simulink library "Load_lib"  (Simulink 8.1)
settings: Solver=ode45  StartTime=0.0  StopTime=10.0  RelTol=1e-3
undefined symbols (not defined in the file): gcbh, sps_rtmsupport, Ts
libraries: powerlib x9, simulink x2, breaker_lib x1, spsPLL3phModel x1, Load_lib x1, powerlib_meascontrol x1
settings Model: Creator=re25624  LastModifiedBy=re25624

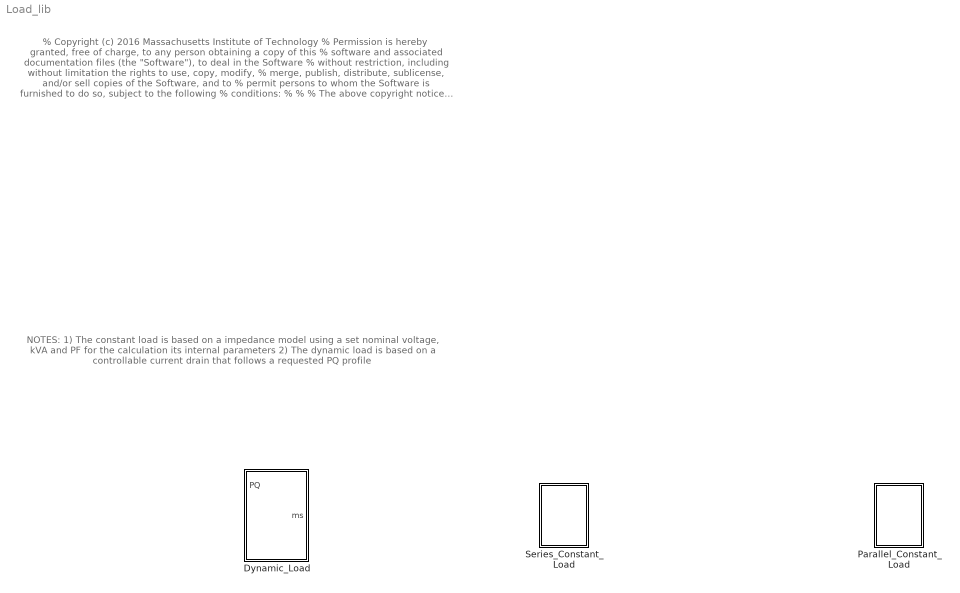
== system Load_lib ==
  note: NOTES:
      | 1) The constant load is based on a impedance model using a set nominal voltage, kVA and PF for the calculation its internal parameters
      |
      | 2) The dynamic load is based on a controllable current drain that follows a requested PQ profile
  note: % Copyright (c) 2016 Massachusetts Institute of Technology
      | % Permission is hereby granted, free of charge, to any person obtaining a copy of this
      | % software and associated documentation files (the "Software"), to deal in the Software
      | % without restriction, including without limitation the rights to use, copy, modify,
      | % merge, publish, distribute, sublicense, and/or sell copies of the Software, and to
      | % permit persons to whom the Software is furnished to do so, subject to the following
      | % conditions:
      | %
      | %
      | % The above copyright notice and this permission notice shall be included in
      | % all copies or substantial portions of the Software.
      | %
      | % THE SOFTWARE IS PROVIDED "AS IS", WITHOUT WARRANTY OF ANY KIND, EXPRESS OR IMPLIED,
      | % INCLUDING BUT NOT LIMITED TO THE WARRANTIES OF MERCHANTABILITY, FITNESS FOR A
      | % PARTICULAR PURPOSE AND NONINFRINGEMENT. IN NO EVENT SHALL THE AUTHORS OR COPYRIGHT
      | % HOLDERS BE LIABLE FOR ANY CLAIM, DAMAGES OR OTHER LIABILITY, WHETHER IN AN ACTION
      | % OF CONTRACT, TORT OR OTHERWISE, ARISING FROM, OUT OF OR IN CONNECTION WITH THE
      | % SOFTWARE OR THE USE OR OTHER DEALINGS IN THE SOFTWARE.
      | %
      | %
      | %%
  Dynamic_Load : Subsystem  mask(Dynamic load){V=460, Ts=Ts}
      mask prompts: V "VRMSLL"; Ts "Simulation Step"
      mask help:
      | The dynamic load model is based on three independent current drains (initialized using nominal voltage) following a terminal voltage and the feed-in kW and kVAr.
      |
      | The current drain of each phase is computed independently permitting unbalanced conditions in the system resulting in unbalanced consumption.
  Parallel_Constant_Load : Subsystem  mask(Static Parallel PQ Load){v=460, kVA=100, pf=0.90}
      mask prompts: v "VRMSLL"
      mask help: The static load model is based on the default Simulink parallel load model. However, a mask was created to permit parametrization using nominal voltage, apparent power, and power factor.
  Series_Constant_Load : Subsystem  mask(Static Series PQ Load){v=460, kVA=100, pf=0.90}
      mask prompts: v "VRMSLL"
      mask help: The static load model is based on the default Simulink parallel load model. However, a mask was created to permit parametrization using nominal voltage, apparent power, and power factor.

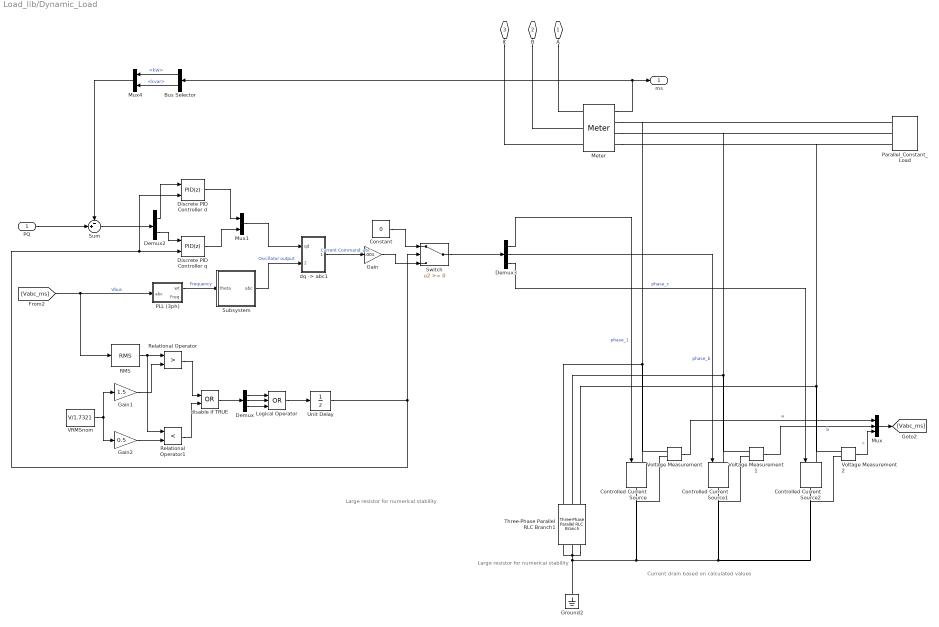
== system Load_lib/Dynamic_Load ==
  note: Large resistor for numerical stability
  note: Current drain based on calculated values
  note: Large resistor for numerical stability
  PQ : Inport
  Bus Selector : BusSelector  OutputSignals=kW,kvar
  Constant : Constant  Value=0
  Controlled Current Source : powerlib/Electrical Sources/Controlled Current Source  Initialize=on  Source_Type=AC  Amplitude=0  Phase=0  Frequency=0  Measurements=None
  Controlled Current Source1 : powerlib/Electrical Sources/Controlled Current Source  Initialize=on  Source_Type=AC  Amplitude=0  Phase=0  Frequency=0  Measurements=None
  Controlled Current Source2 : powerlib/Electrical Sources/Controlled Current Source  Initialize=on  Source_Type=AC  Amplitude=0  Phase=0  Frequency=0  Measurements=None
  Demux : Demux  Outputs=3
  Demux2 : Demux  Outputs=2
  Demux3 : Demux  Outputs=3
  Discrete PID Controller d : simulink/Continuous/PID Controller  Controller=PID  TimeDomain=Discrete-time  SampleTime=Ts  IntegratorMethod=Forward Euler  FilterMethod=Forward Euler  Form=Parallel  P=0  I=2000  D=0  N=100  InitialConditionSource=internal  InitialConditionForIntegrator=0  InitialConditionForFilter=0  ExternalReset=level  LimitOutput=off  UpperSaturationLimit=inf  LowerSaturationLimit=-inf  LinearizeAsGain=off  AntiWindupMode=none  Kb=1  TrackingMode=off  Kt=1  PParamMin=[]  PParamMax=[]  IParamMin=[]  IParamMax=[]  DParamMin=[]  DParamMax=[]  NParamMin=[]  NParamMax=[]  KbParamMin=[]  KbParamMax=[]  KtParamMin=[]  KtParamMax=[]  POutMin=[]  POutMax=[]  IOutMin=[]  IOutMax=[]  DOutMin=[]  DOutMax=[]  NOutMin=[]  NOutMax=[]  KbOutMin=[]  KbOutMax=[]  KtOutMin=[]  KtOutMax=[]  IntegratorOutMin=[]  IntegratorOutMax=[]  FilterOutMin=[]  FilterOutMax=[]  SumOutMin=[]  SumOutMax=[]  SumI1OutMin=[]  SumI1OutMax=[]  SumI2OutMin=[]  SumI2OutMax=[]  SumI3OutMin=[]  SumI3OutMax=[]  SumDOutMin=[]  SumDOutMax=[]  SaturationOutMin=[]  SaturationOutMax=[]  IntegratorContinuousStateAttributes=''  IntegratorStateMustResolveToSignalObject=off  IntegratorRTWStateStorageClass=Auto  FilterContinuousStateAttributes=''  FilterStateMustResolveToSignalObject=off  FilterRTWStateStorageClass=Auto
  Discrete PID Controller q : simulink/Continuous/PID Controller  Controller=PID  TimeDomain=Discrete-time  SampleTime=Ts  IntegratorMethod=Forward Euler  FilterMethod=Forward Euler  Form=Parallel  P=0  I=-2000  D=0  N=100  InitialConditionSource=internal  InitialConditionForIntegrator=0  InitialConditionForFilter=0  ExternalReset=level  LimitOutput=off  UpperSaturationLimit=inf  LowerSaturationLimit=-inf  LinearizeAsGain=off  AntiWindupMode=none  Kb=1  TrackingMode=off  Kt=1  PParamMin=[]  PParamMax=[]  IParamMin=[]  IParamMax=[]  DParamMin=[]  DParamMax=[]  NParamMin=[]  NParamMax=[]  KbParamMin=[]  KbParamMax=[]  KtParamMin=[]  KtParamMax=[]  POutMin=[]  POutMax=[]  IOutMin=[]  IOutMax=[]  DOutMin=[]  DOutMax=[]  NOutMin=[]  NOutMax=[]  KbOutMin=[]  KbOutMax=[]  KtOutMin=[]  KtOutMax=[]  IntegratorOutMin=[]  IntegratorOutMax=[]  FilterOutMin=[]  FilterOutMax=[]  SumOutMin=[]  SumOutMax=[]  SumI1OutMin=[]  SumI1OutMax=[]  SumI2OutMin=[]  SumI2OutMax=[]  SumI3OutMin=[]  SumI3OutMax=[]  SumDOutMin=[]  SumDOutMax=[]  SaturationOutMin=[]  SaturationOutMax=[]  IntegratorContinuousStateAttributes=''  IntegratorStateMustResolveToSignalObject=off  IntegratorRTWStateStorageClass=Auto  FilterContinuousStateAttributes=''  FilterStateMustResolveToSignalObject=off  FilterRTWStateStorageClass=Auto
  Gain : Gain  Gain=.001
  Gain1 : Gain  Gain=1.5
  Gain2 : Gain  Gain=0.5
  Ground2 : powerlib/Elements/Ground  LConnTagsString=a
  Logical Operator : Logic  Operator=OR  Inputs=3  AllPortsSameDT=off  OutDataTypeStr=boolean
  Meter : breaker_lib/Meter  Ts=Ts
  Mux : Mux  Inputs=3
  Mux1 : Mux  Inputs=2
  Mux4 : Mux  Inputs=2
  PLL (3ph) : Subsystem  DialogController=POWERSYS.PowerSysDialog  mask(PLL (3ph)){Fmin=45, Par_Init=[0, 60], ParK=[180, 5000, 1], TcD=1e-4, MaxRateChangeFreq=12, FilterCutOffFreq=25, Ts=Ts, AGC=on}
      mask prompts: Fmin "Minimum frequency (Hz):"; Par_Init "Initial inputs [ Phase (degrees), Frequency (Hz) ]:"; ParK "Regulator gains [ Kp, Ki, Kd ]:"; TcD "Time constant for derivative action (s):"; MaxRateChangeFreq "Maximum rate of change of frequency (Hz/s):"; FilterCutOffFreq "Filter cut-off frequency for frequency measurement (Hz):"; Ts "Sample time:"; AGC "Enable automatic gain control"
      mask help:
      | This Phase Locked Loop (PLL) system can be used  to synchronize on a set of variable frequency, three-phase sinusoidal signals. If the Automatic Gain Control is enabled, the input (phase error) of the PLL regulator is scaled according to the input signals magnitude.
      |
      | For optimal performance, set regulator gains [ Kp Ki  Kd ] = [ 180  3200  1 ] and check the Enable Automatic Gain Control parameter.
      |
      | Input : Vector containing the normalized three-phase signals [Va Vb Vc]
      | Output 1:  Measured frequency (Hz) = w/(2pi)
      | Output 2:  Ramp w.t varying between  0 and 2*pi, synchronized on zero crossings of the fundamental (positive-sequence) of phase A.
      mask init:
      | block=gcb;
      | [WantBlockChoice,Ts,sps] = powericon('PLL3phInit',block,Fmin,Par_Init,ParK,TcD, MaxRateChangeFreq, FilterCutOffFreq, AGC,Ts);
      | powericon('SetInternalModels','set',block,WantBlockChoice);
      settings: OpenFcn=power_openblockproxy();
      mask Help: helpview(psbhelp);
  Parallel_Constant_Load : Load_lib/Parallel_Constant_Load  v=V  kVA=5  pf=0.9
  RMS : powerlib_meascontrol/Measurements/RMS  TrueRMS=on  Freq=60  RMSInit=120  Ts=Ts
  Relational Operator : RelationalOperator  Operator=>  OutDataTypeStr=boolean
  Relational Operator1 : RelationalOperator  Operator=<  OutDataTypeStr=boolean
  Subsystem : Subsystem
  Sum : Sum  Inputs=-+|
  Switch : Switch
  Three-Phase Parallel RLC Branch1 : powerlib/Elements/Three-Phase Parallel RLC Branch  LConnTagsString=A|B|C  RConnTagsString=A|B|C  BranchType=RLC  Resistance=1e6  Inductance=inf  Capacitance=0  Measurements=None
  Unit Delay : UnitDelay  SampleTime=-1
  VRMSnom : Constant  Value=V/1.7321  SampleTime=Ts
  Voltage Measurement : powerlib/Measurements/Voltage Measurement  PhasorSimulation=off  OutputType=Complex  PSBequivalent=0
  Voltage Measurement1 : powerlib/Measurements/Voltage Measurement  PhasorSimulation=off  OutputType=Complex  PSBequivalent=0
  Voltage Measurement2 : powerlib/Measurements/Voltage Measurement  PhasorSimulation=off  OutputType=Complex  PSBequivalent=0
  disable if TRUE : Logic  Operator=OR  AllPortsSameDT=off  OutDataTypeStr=boolean
  "dq -> abc1" : Subsystem
  A : PMIOPort  Port=1  Side=Left
  B : PMIOPort  Port=2  Side=Left
  C : PMIOPort  Port=3  Side=Left
  ms : Outport
  wires:
  Voltage Measurement/1 -> Mux/1  "a"
  Voltage Measurement1/1 -> Mux/2  "b"
  Voltage Measurement2/1 -> Mux/3  "c"
  Mux/1 -> [Vabc_ms]
  Demux3/1 -> Controlled Current Source/1  "phase_1"
  Demux3/2 -> Controlled Current Source1/1  "phase_b"
  Demux3/3 -> Controlled Current Source2/1  "phase_c"
  Switch/1 -> Demux3/1
  Gain/1 -> Switch/3
  PLL (3ph)/1(wt) -> Subsystem/1(theta)  "Frequency"
  Subsystem/1(abc) -> "dq -> abc1"/2(Vabc)  "Oscillator output"
  Mux4/1 -> Sum/1
  Discrete PID Controller q/1 -> Mux1/2
  Discrete PID Controller d/1 -> Mux1/1
  Mux1/1 -> "dq -> abc1"/1(qd)
  Demux2/2 -> Discrete PID Controller q/1
  Demux2/1 -> Discrete PID Controller d/1
  Sum/1 -> Demux2/1
  "dq -> abc1"/1(abc) -> Gain/1  "Current Command_abc"
  [Vabc_ms] -> PLL (3ph)/1(abc), RMS/1  "Vbus"
  PQ/1 -> Sum/2
  RMS/1 -> Relational Operator/1, Relational Operator1/1
  VRMSnom/1 -> Gain2/1, Gain1/1
  Gain1/1 -> Relational Operator/2
  Gain2/1 -> Relational Operator1/2
  Relational Operator/1 -> disable if TRUE/1
  Relational Operator1/1 -> disable if TRUE/2
  disable if TRUE/1 -> Demux/1
  Constant/1 -> Switch/1
  Unit Delay/1 -> Discrete PID Controller q/2, Discrete PID Controller d/2, Switch/2
  Demux/1 -> Logical Operator/1
  Demux/2 -> Logical Operator/2
  Demux/3 -> Logical Operator/3
  Logical Operator/1 -> Unit Delay/1
  Bus Selector/1 -> Mux4/1  "<kW>"
  Bus Selector/2 -> Mux4/2  "<kvar>"
  Meter/1 -> ms/1, Bus Selector/1
  connections:
  Voltage Measurement/LConn1 -- Controlled Current Source/LConn1 -- Meter/RConn1 -- Parallel_Constant_Load/RConn1 -- Three-Phase Parallel RLC Branch1/RConn1
  Voltage Measurement1/LConn1 -- Controlled Current Source1/LConn1 -- Parallel_Constant_Load/RConn2 -- Meter/RConn2 -- Three-Phase Parallel RLC Branch1/RConn2
  Voltage Measurement2/LConn1 -- Controlled Current Source2/LConn1 -- Parallel_Constant_Load/RConn3 -- Meter/RConn3 -- Three-Phase Parallel RLC Branch1/RConn3
  Voltage Measurement2/LConn2 -- Controlled Current Source2/RConn1 -- Three-Phase Parallel RLC Branch1/LConn1 -- Three-Phase Parallel RLC Branch1/LConn2 -- Three-Phase Parallel RLC Branch1/LConn3 -- Ground2/LConn1 -- Voltage Measurement/LConn2 -- Controlled Current Source/RConn1 -- Voltage Measurement1/LConn2 -- Controlled Current Source1/RConn1
  A/RConn1 -- Meter/LConn1
  B/RConn1 -- Meter/LConn2
  C/RConn1 -- Meter/LConn3

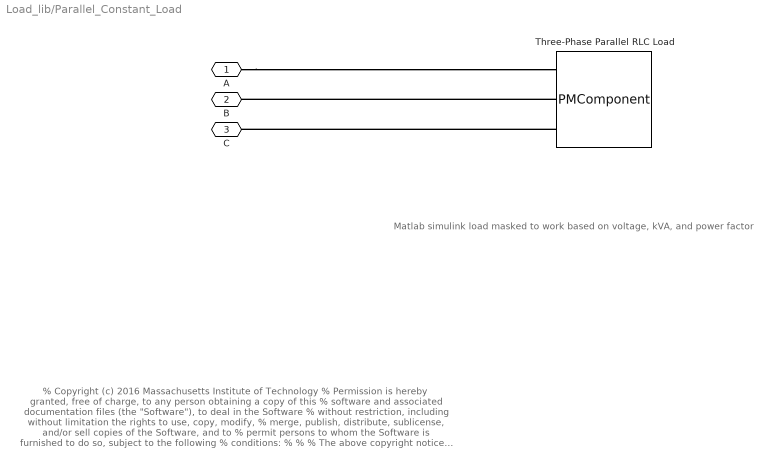
== system Load_lib/Parallel_Constant_Load ==
  note: Matlab simulink load masked to work based on voltage, kVA, and power factor
  note: % Copyright (c) 2016 Massachusetts Institute of Technology
      | % Permission is hereby granted, free of charge, to any person obtaining a copy of this
      | % software and associated documentation files (the "Software"), to deal in the Software
      | % without restriction, including without limitation the rights to use, copy, modify,
      | % merge, publish, distribute, sublicense, and/or sell copies of the Software, and to
      | % permit persons to whom the Software is furnished to do so, subject to the following
      | % conditions:
      | %
      | %
      | % The above copyright notice and this permission notice shall be included in
      | % all copies or substantial portions of the Software.
      | %
      | % THE SOFTWARE IS PROVIDED "AS IS", WITHOUT WARRANTY OF ANY KIND, EXPRESS OR IMPLIED,
      | % INCLUDING BUT NOT LIMITED TO THE WARRANTIES OF MERCHANTABILITY, FITNESS FOR A
      | % PARTICULAR PURPOSE AND NONINFRINGEMENT. IN NO EVENT SHALL THE AUTHORS OR COPYRIGHT
      | % HOLDERS BE LIABLE FOR ANY CLAIM, DAMAGES OR OTHER LIABILITY, WHETHER IN AN ACTION
      | % OF CONTRACT, TORT OR OTHERWISE, ARISING FROM, OUT OF OR IN CONNECTION WITH THE
      | % SOFTWARE OR THE USE OR OTHER DEALINGS IN THE SOFTWARE.
      | %
      | %
      | %%
  Three-Phase Parallel RLC Load : PMComponent  DialogController=POWERSYS.PowerSysDialog  LoadFcn=sps_rtmsupport('LoadFcn',gcbh);  StartFcn=sps_rtmsupport('StartFcn',gcbh);  StopFcn=sps_rtmsupport('StopFcn',gcbh);  PhysicalDomain=powersysdomain  LeftPortType=p1  RightPortType=p1  LConnTagsString=A|B|C  mask(Three-Phase Parallel RLC Load){Configuration=Y (grounded), NominalVoltage=v, NominalFrequency=60, ActivePower=kVA*1E3*pf, InductivePower=kVA*1E3*sqrt(1-pf^2), CapacitivePower=0, Measurements=None, LoadType=constant Z}
      mask prompts: NominalVoltage "Nominal phase-to-phase voltage Vn (Vrms)"; NominalFrequency "Nominal frequency fn (Hz):"; ActivePower "Active power P (W):"; InductivePower "Inductive reactive Power QL (positive var):"; CapacitivePower "Capacitive reactive power Qc (negative var):"; LoadType "Load type"
      mask help: Implements a three-phase parallel RLC load.
      mask init:
      | [s1,s2,s3,s4,r1,r2,l1,l2,c1,c2,c3,c4,x1,x2,x3,x4] = powericon('Parallel RLC Load',ActivePower,InductivePower,CapacitivePower);
      | ground = Configuration==1;
      | neutral = Configuration==3;
      | power_initmask();
      settings: AttributesFormatString=\n  CopyFcn=sps_rtmsupport('CopyFcn',gcbh);  DeleteFcn=sps_rtmsupport('DeleteFcn',gcbh);  UndoDeleteFcn=sps_rtmsupport('UndoDeleteFcn',gcbh);  ModelCloseFcn=sps_rtmsupport('ModelCloseFcn',gcbh);  PreSaveFcn=sps_rtmsupport('PreSaveFcn',gcbh);  PostSaveFcn=sps_rtmsupport('PostSaveFcn',gcbh);  NameChangeFcn=sps_rtmsupport('NameChangeFcn',gcbh);  PreCopyFcn=sps_rtmsupport('PreCopyFcn',gcbh);  OpenFcn=sps_rtmsupport('OpenFcn',gcbh, [1 7 8]);  CloseFcn=sps_rtmsupport('CloseFcn',gcbh);  PreDeleteFcn=sps_rtmsupport('PreDeleteFcn',gcbh);
      mask Help: helpview(psbhelp);
      mask TypeOptions Configuration: Y (grounded) | Y (floating) | Y (neutral) | Delta
      mask Callback Configuration: powericon('psbcallbacks',gcb,'Three-Phase Parallel RLC Load');
      mask TypeOptions Measurements: None | Branch voltages | Branch currents | Branch voltages and currents
      mask TypeOptions LoadType: constant Z | constant PQ
      mask Display:
      | plot(s1-50,s2,s3+30,s4,r1,r2,l1,l2,c1,c2,c3,c4,x1,x2,x3,x4)
      | 
      | plot( ground*[s3,s3],  ground*[-s2/4,s2/4])
      | plot( ground*[s3+10,s3+10], ground*[-s2/6,s2/6])
      | plot( ground*[s3+20,s3+20], ground*[-s2/10,s2/10])
      | 
      | plot( neutral*[ s3,s3+30], neutral*[0,0])
      | port_label('LConn', 1, 'A')
      | port_label('LConn', 2, 'B')
      | port_label('LConn', 3, 'C')
  A : PMIOPort  Port=1  Side=Right
  B : PMIOPort  Port=2  Side=Right
  C : PMIOPort  Port=3  Side=Right
  connections:
  Three-Phase Parallel RLC Load/LConn2 -- B/RConn1
  Three-Phase Parallel RLC Load/LConn3 -- C/RConn1
  A/RConn1 -- Three-Phase Parallel RLC Load/LConn1

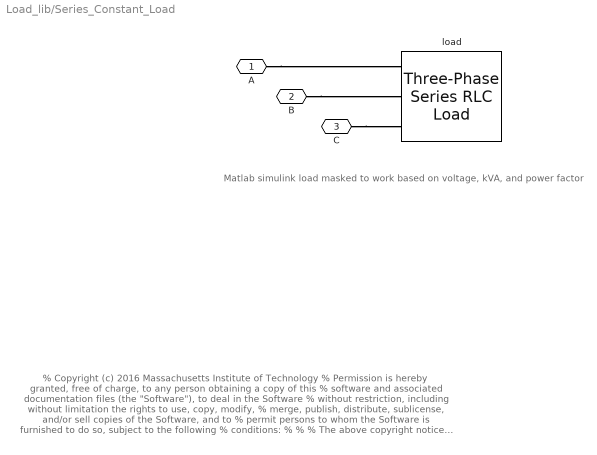
== system Load_lib/Series_Constant_Load ==
  note: Matlab simulink load masked to work based on voltage, kVA, and power factor
  note: % Copyright (c) 2016 Massachusetts Institute of Technology
      | % Permission is hereby granted, free of charge, to any person obtaining a copy of this
      | % software and associated documentation files (the "Software"), to deal in the Software
      | % without restriction, including without limitation the rights to use, copy, modify,
      | % merge, publish, distribute, sublicense, and/or sell copies of the Software, and to
      | % permit persons to whom the Software is furnished to do so, subject to the following
      | % conditions:
      | %
      | %
      | % The above copyright notice and this permission notice shall be included in
      | % all copies or substantial portions of the Software.
      | %
      | % THE SOFTWARE IS PROVIDED "AS IS", WITHOUT WARRANTY OF ANY KIND, EXPRESS OR IMPLIED,
      | % INCLUDING BUT NOT LIMITED TO THE WARRANTIES OF MERCHANTABILITY, FITNESS FOR A
      | % PARTICULAR PURPOSE AND NONINFRINGEMENT. IN NO EVENT SHALL THE AUTHORS OR COPYRIGHT
      | % HOLDERS BE LIABLE FOR ANY CLAIM, DAMAGES OR OTHER LIABILITY, WHETHER IN AN ACTION
      | % OF CONTRACT, TORT OR OTHERWISE, ARISING FROM, OUT OF OR IN CONNECTION WITH THE
      | % SOFTWARE OR THE USE OR OTHER DEALINGS IN THE SOFTWARE.
      | %
      | %
      | %%
  load : powerlib/Elements/Three-Phase Series RLC Load  LConnTagsString=A|B|C  Configuration=Y (grounded)  NominalVoltage=v  NominalFrequency=60  ActivePower=kVA*1E3*pf  InductivePower=kVA*1E3*sqrt(1-pf^2)  CapacitivePower=0  Measurements=None  LoadType=constant Z
  A : PMIOPort  Port=1  Side=Left
  B : PMIOPort  Port=2  Side=Left
  C : PMIOPort  Port=3  Side=Left
  connections:
  A/RConn1 -- load/LConn1
  B/RConn1 -- load/LConn2
  C/RConn1 -- load/LConn3

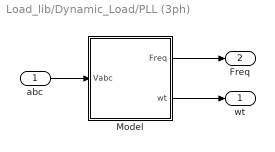
== system Load_lib/Dynamic_Load/PLL (3ph) ==
  abc : Inport  PortDimensions=3  SampleTime=Ts
  Model : Subsystem  BlockChoice=Discrete
      settings: AttributesFormatString=%<BlockChoice>  TemplateBlock=spsPLL3phModel/Model  MemberBlocks=Continuous,Discrete
  wt : Outport  SampleTime=Ts
  Freq : Outport  Port=2  SampleTime=Ts
  wires:
  Model/2(wt) -> wt/1
  Model/1(Freq) -> Freq/1
  abc/1 -> Model/1(Vabc)

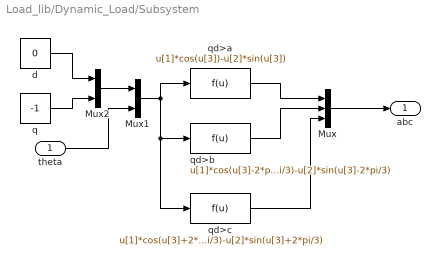
== system Load_lib/Dynamic_Load/Subsystem ==
  theta : Inport  OutDataTypeStr=double  PortDimensions=1
  Mux : Mux  Inputs=3
  Mux1 : Mux  Inputs=2
  Mux2 : Mux  Inputs=2
  d : Constant  Value=0
  q : Constant  Value=-1
  qd>a : Fcn  Expr=u[1]*cos(u[3])-u[2]*sin(u[3])
  qd>b : Fcn  Expr=u[1]*cos(u[3]-2*pi/3)-u[2]*sin(u[3]-2*pi/3)
  qd>c : Fcn  Expr=u[1]*cos(u[3]+2*pi/3)-u[2]*sin(u[3]+2*pi/3)
  abc : Outport  OutDataTypeStr=double  PortDimensions=3
  wires:
  Mux/1 -> abc/1
  qd>b/1 -> Mux/2
  qd>c/1 -> Mux/3
  theta/1 -> Mux1/2
  Mux1/1 -> qd>c/1, qd>b/1, qd>a/1
  qd>a/1 -> Mux/1
  d/1 -> Mux2/1
  q/1 -> Mux2/2
  Mux2/1 -> Mux1/1

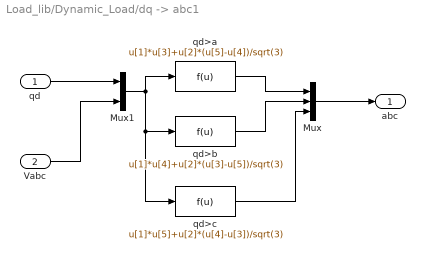
== system Load_lib/Dynamic_Load/dq -> abc1 ==
  qd : Inport  OutDataTypeStr=double  PortDimensions=2
  Vabc : Inport  Port=2  PortDimensions=3
  Mux : Mux  Inputs=3
  Mux1 : Mux  Inputs=2
  qd>a : Fcn  Expr=u[1]*u[3]+u[2]*(u[5]-u[4])/sqrt(3)
  qd>b : Fcn  Expr=u[1]*u[4]+u[2]*(u[3]-u[5])/sqrt(3)
  qd>c : Fcn  Expr=u[1]*u[5]+u[2]*(u[4]-u[3])/sqrt(3)
  abc : Outport  OutDataTypeStr=double  PortDimensions=3
  wires:
  Mux/1 -> abc/1
  Vabc/1 -> Mux1/2
  qd>a/1 -> Mux/1
  Mux1/1 -> qd>a/1, qd>b/1, qd>c/1
  qd>c/1 -> Mux/3
  qd/1 -> Mux1/1
  qd>b/1 -> Mux/2

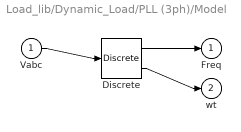
== system Load_lib/Dynamic_Load/PLL (3ph)/Model ==
  Vabc : Inport
  Discrete : spsPLL3phModel/Discrete
  Freq : Outport
  wt : Outport  Port=2
  wires:
  Discrete/2 -> wt/1
  Discrete/1 -> Freq/1
  Vabc/1 -> Discrete/1
